simulink model "mavsim_chap3"  (R2024a)
settings: Solver=ode45  StartTime=0.0  StopTime=30  RelTol=1e-3  EnableMultiTasking=on
InitFcn:
  | addpath('../chap2')
  | addpath('../parameters/')
  | aerosonde_parameters
undefined symbols (not defined in the file): drawAircraft, plotmavstatevariables
libraries: simulink x6
settings Model: Creator=beard  LastModifiedBy=Admin
settings SolverCC: AlgebraicLoopSolver=TrustRegion
settings DataIOCC: LimitDataPoints=on  SaveFormat=Array  SignalLoggingSaveFormat=ModelDataLogs  ReturnWorkspaceOutputs=off
settings OptimizationCC: ExpressionDepthLimit=2147483647  InitFltsAndDblsToZero=on  LifeSpan=inf
settings DebuggingCC: UnderspecifiedInitializationDetection=Classic  MergeDetectMultiDrivingBlocksExec=none  SolverPrmCheckMsg=warning  FcnCallInpInsideContextMsg=warning  UnconnectedInputMsg=warning  UnconnectedOutputMsg=warning  UnconnectedLineMsg=warning  AllowSymbolicDim=off  StateNameClashWarn=warning  SFUnexpectedBacktrackingDiag=warning  SFNoUnconditionalDefaultTransitionDiag=warning  SFExecutionAtInitializationDiag=none  ArithmeticOperatorsInVariantConditions=warning
settings HardwareCC: ProdBitPerPointer=32  ProdBitPerSizeT=32  ProdBitPerPtrDiffT=32  ProdLargestAtomicFloat=None  ProdIntDivRoundTo=Undefined  ProdEndianess=Unspecified  ProdWordSize=32  ProdHWDeviceType=32-bit Generic
settings ModelReferenceCC: EnableRefExpFcnMdlSchedulingChecks=on  PropagateSignalLabelsOutOfModel=off
settings SFSimCC: SimUseLocalCustomCode=off  CustomCodeUndefinedFunction=UseInterfaceOnly
settings RTWCC: RTWUseLocalCustomCode=off  GPUComputeCapability=3.5
settings CodeAppCC: StateflowObjectComments=on
settings GRTTargetCC: TargetLangStandard=C89/C90 (ANSI)  CombineOutputUpdateFcns=off  GRTInterface=on
settings ConfigComp: CovMetricSettings=dw  CovSaveCumulativeToWorkspaceVar=on  CovSaveSingleToWorkspaceVar=on  CovExternalEMLEnable=off  CovSFcnEnable=off

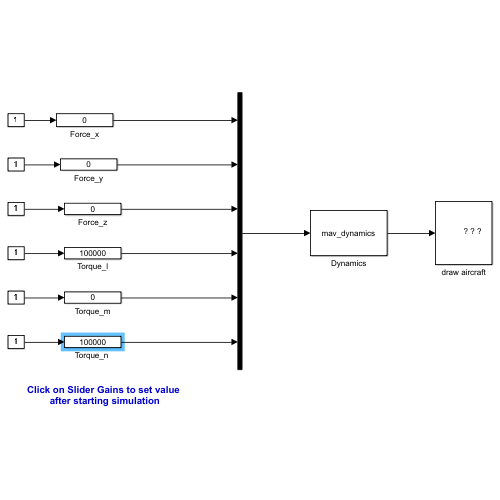
[thumbnail: Simulink's stored preview of the top-level diagram]
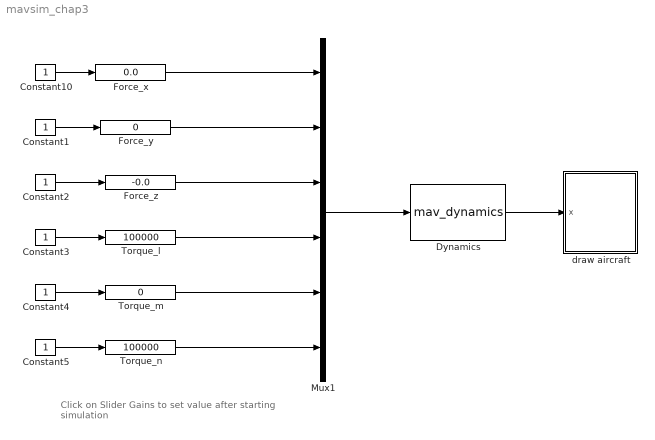
== system mavsim_chap3 ==
  note: Click on Slider Gains to set value
      | after starting simulation
  Constant{1..5,10} (6 alike) : Constant
  Dynamics : S-Function  FunctionName=mav_dynamics  Parameters=MAV  SFunctionDeploymentMode=off  EnableBusSupport=off
  Force_x : simulink/Math Operations/Slider Gain  gain=0.0  low=-1  high=1
  Force_y : simulink/Math Operations/Slider Gain  gain=0  low=-99999999  high=99999999
  Force_z : simulink/Math Operations/Slider Gain  gain=-0.0  low=-1  high=1
  Mux1 : Mux  Inputs=6
  Torque_l : simulink/Math Operations/Slider Gain  gain=100000  low=-999999  high=999999
  Torque_m : simulink/Math Operations/Slider Gain  gain=0  low=-0.1  high=0.1
  "Torque_n " : simulink/Math Operations/Slider Gain  gain=100000  low=-999999  high=999999
  draw aircraft : Subsystem
      mask Display: image(imread('../chap2/tv.jpg'))
  wires:
  Constant5/1 -> "Torque_n "/1
  Constant10/1 -> Force_x/1
  Constant1/1 -> Force_y/1
  Constant2/1 -> Force_z/1
  Dynamics/1 -> draw aircraft/1(x)
  Force_z/1 -> Mux1/3
  Force_y/1 -> Mux1/2
  Force_x/1 -> Mux1/1
  "Torque_n "/1 -> Mux1/6
  Constant4/1 -> Torque_m/1
  Torque_m/1 -> Mux1/5
  Constant3/1 -> Torque_l/1
  Torque_l/1 -> Mux1/4
  Mux1/1 -> Dynamics/1

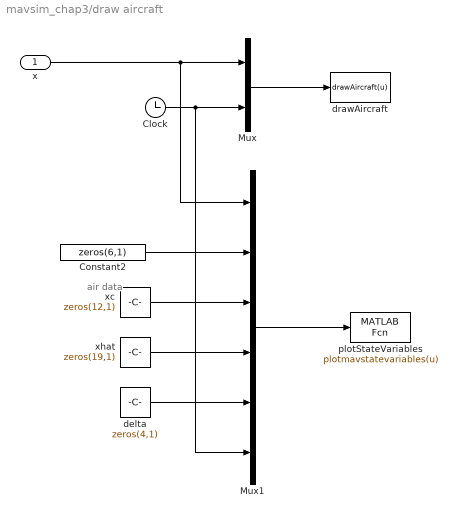
== system mavsim_chap3/draw aircraft ==
  note: air data
  x : Inport
  Clock : Clock
  Constant2 : Constant  Value=zeros(6,1)
  Mux : Mux  Inputs=2
  Mux1 : Mux  Inputs=6
  delta : Constant  Value=zeros(4,1)
  drawAircraft : MATLABFcn  MATLABFcn=drawAircraft(u)  OutputDimensions=0  SampleTime=0.1
  plotStateVariables : MATLABFcn  MATLABFcn=plotmavstatevariables(u)  OutputDimensions=0  SampleTime=0.1
  xc : Constant  Value=zeros(12,1)
  xhat : Constant  Value=zeros(19,1)
  wires:
  Mux/1 -> drawAircraft/1
  x/1 -> Mux/1, Mux1/1
  Clock/1 -> Mux/2, Mux1/6
  Mux1/1 -> plotStateVariables/1
  xhat/1 -> Mux1/4
  xc/1 -> Mux1/3
  delta/1 -> Mux1/5
  Constant2/1 -> Mux1/2
